simulink model "modelSim"  (R2019a)
settings: Solver=VariableStepAuto  StartTime=0.0  StopTime=10.0  RelTol=1e-3
InitFcn:
  | modelSimVar
values from neighbouring files (symbols this model uses):
  setV_Norm = SamplesStepping.mVel    [A02_FreeMotSimVar.m]    (also in A03_BoldMotSimVar.m; Motor0_255_est.m = Samples(1:bfStart,3); MotorStepping.m = Samples(:,3); modelSimVar.m = Samples_10ms(1:850,3))
  Ts = test.Time(2)    [A02_FreeMotSimVar.m]    (also in A03_BoldMotSimVar.m; Motor.m = floor(16000*1000*timeWanted/1024)*0.064*0.001; Motor0_255_est.m = floor(16000*1000*timeWanted/1024)*0.064*0.001; MotorMultipleCalc.m = floor(16000*1000*timeWanted/1024)*0.064*0.001)
  v0 = 0    [A02_FreeMotSimVar.m]    (also in A03_BoldMotSimVar.m; Motor0_255_est.m; MotorStepping.m; modelSimVar.m)
libraries: dspsrcs4 x2
settings Model: Creator=alfyhack  LastModifiedBy=alfyhack

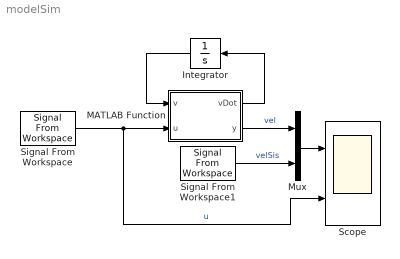
== system modelSim ==
  Integrator : Integrator  InitialCondition=v0
  MATLAB Function : MATLAB Function  TreatAsAtomicUnit=on
  Mux : Mux  Inputs=2
  Scope : Scope  NumInputPorts=2
  Signal From Workspace : dspsrcs4/Signal From Workspace  X=setU_Norm  Ts=Ts  nsamps=1  OutputAfterFinalValue=Setting to zero  ignoreOrWarnInputAndFrameLengths=off  OutputFrames=off
  Signal From Workspace1 : dspsrcs4/Signal From Workspace  X=[[0] [setV_Norm']]  Ts=Ts  nsamps=1  OutputAfterFinalValue=Setting to zero  ignoreOrWarnInputAndFrameLengths=off  OutputFrames=off
  wires:
  MATLAB Function/1(vDot) -> Integrator/1
  Integrator/1 -> MATLAB Function/1(v)
  Signal From Workspace/1 -> Scope/2, MATLAB Function/2(u)  "u"
  MATLAB Function/2(y) -> Mux/1  "vel"
  Signal From Workspace1/1 -> Mux/2  "velSis"
  Mux/1 -> Scope/1

== matlab function modelSim/MATLAB Function ==
  data: v input; vDot output; u input; y output
function [vDot,y] = motor(v,u)
% u= % pwm al motore

coder.extrinsic('evalin', 'assignin')

ka = 0;                  % Needed in order to set variable class correctly
ka = evalin('base','ka'); % Read value from workspace

rhoAtt = 0;                  % Needed in order to set variable class correctly
rhoAtt = evalin('base','rhoAtt'); % Read value from workspace

rhoAttDyn = 0;
rhoAttDyn = evalin('base','rhoAttDyn'); % Read value from workspace

rhoMag = 0;                  % Needed in order to set variable class correctly
rhoMag = evalin('base','rhoMag'); % Read value from workspace

rho = 0;                  % Needed in order to set variable class correctly
rho = evalin('base','rho'); % Read value from workspace

velmax = 0;
velmax = evalin('base','velmax'); % Read value from workspace


% if(abs(v)>0.001)
%     vDot = -(rhoMag*abs(u)+0.23 + rhoAttDyn/abs(v))*v + ka*u;
% else
%     vDot = -(rhoMag*abs(u)+0.23 )*v + ka*u;
% end

if(abs(v)>0.001)
    vDot = -((rho)*abs(u)+ 0.20 + (rhoAttDyn*0.9)/abs(v))*v + ka*u;
else
    vDot = -(rho*abs(u)+0.23 )*v + ka*u;
end
y=v;
end
